simulink model "CanBusRagnar2020"  (R2021a)
settings: Solver=VariableStepAuto  StartTime=0.0  StopTime=10.0  RelTol=1e-3
model workspace (MAT data in the model file):
  A = [0  0  0  0  1  0  0  0; 0  0  0  0  0  1  0  0; 0  0  0  0  0  0  1  0; 0  0  0  0  0  0  0  1; 0  0  0  0  0  0  0  0; 0  0  0  0  0  0  0  0; 0  0  0  0  0  0  0  0; 0  0  0  0  0  0  0  0]
  Acl = [0  0  0  0  1  0  0  0  0  0  0  0  0  0  0  0; 0  0  0  0  0  1  0  0  0  0  0  0  0  0  0  0; 0  0  0  0  0  0  1  0  0  0  0  0  0  0  0  0; 0  0  0  0  0  0  0  1  0  0  0  0  0  0  0  0; 0  0  0  0  0  0  0  0  -1.14285714286  0  0  0  -2.14285714286  0  0  0; 0  0  0  0  0  0  0  0  0  -2.69387755102  0  0  0  -3.28571428571  0  0; 0  0  0  0  0  0  0  0  0  0  -2.38775510204  0  0  0  -3.14285714286  0; 0  0  0  0  0  0  0  0  0  0  0  -2.85714285714  0  0  0  -3.42857142857; 8.14285714286  0  0  0  0  0  0  0  -8.14285714286  0  0  0  1  0  0  0; 0  9.28571428571  0  0  0  0  0  0  0  -9.28571428571  0  0  0  1  0  0; 0  0  9.14285714286  0  0  0  0  0  0  0  -9.14285714286  0  0  0  1  0; 0  0  0  9.42857142857  0  0  0  0  0  0  0  -9.42857142857  0  0  0  1; 16.5714285714  0  0  0  0  0  0  0  -17.7142857143  0  0  0  -2.14285714286  0  0  0; 0  21.5510204082  0  0  0  0  0  0  0  -24.2448979592  0  0  0  -3.28571428571  0  0; 0  0  20.8163265306  0  0  0  0  0  0  0  -23.2040816327  0  0  0  -3.14285714286  0; 0  0  0  22.1428571429  0  0  0  0  0  0  0  -25  0  0  0  -3.42857142857]
  Ak_mimo = [-8.14285714286  0  0  0  1  0  0  0; 0  -9.28571428571  0  0  0  1  0  0; 0  0  -9.14285714286  0  0  0  1  0; 0  0  0  -9.42857142857  0  0  0  1; -17.7142857143  0  0  0  -2.14285714286  0  0  0; 0  -24.2448979592  0  0  0  -3.28571428571  0  0; 0  0  -23.2040816327  0  0  0  -3.14285714286  0; 0  0  0  -25  0  0  0  -3.42857142857]
  Ar = [0  0  0  0  1  0  0  0; 0  0  0  0  0  1  0  0; 0  0  0  0  0  0  1  0; 0  0  0  0  0  0  0  1; 0  0  0  0  0  0  0  0; 0  0  0  0  0  0  0  0; 0  0  0  0  0  0  0  0; 0  0  0  0  0  0  0  0]
  Aza = [-8.14285714286  0  0  0  1  0  0  0; 0  -9.28571428571  0  0  0  1  0  0; 0  0  -9.14285714286  0  0  0  1  0; 0  0  0  -9.42857142857  0  0  0  1; -17.7142857143  0  0  0  -2.14285714286  0  0  0; 0  -24.2448979592  0  0  0  -3.28571428571  0  0; 0  0  -23.2040816327  0  0  0  -3.14285714286  0; 0  0  0  -25  0  0  0  -3.42857142857]
  B = [0  0  0  0; 0  0  0  0; 0  0  0  0; 0  0  0  0; 0.78125  0  0  0; 0  0.78125  0  0; 0  0  0.78125  0; 0  0  0  2180]
  BScal = [0  0  0  0  0  0  0  0; 0  0  0  0  0  0  0  0; 0  0  0  0  0  0  0  0; 0  0  0  0  0  0  0  0; 0  0  0  0  0.78125  0  0  0; 0  0  0  0  0  0.78125  0  0; 0  0  0  0  0  0  0.78125  0; 0  0  0  0  0  0  0  2180]
  B_tilde_cl = [0  0  0  0; 0  0  0  0; 0  0  0  0; 0  0  0  0; 0.78125  0  0  0; 0  0.78125  0  0; 0  0  0.78125  0; 0  0  0  2180; 0.385570788906  0  0  0; 0  0.206011164513  0  0; 0  0  0.222133260428  0; 0  0  0  542.533936652; 2.03394557925  0  0  0; 0  1.56343339307  0  0; 0  0  1.60680460084  0; 0  0  0  4271.22171946]
  Bcl = [0  0  0  0; 0  0  0  0; 0  0  0  0; 0  0  0  0; 4.41904761905  0  0  0; 0  8.3179377014  0  0; 0  0  7.61096938775  0; 0  0  0  8.68347338936; 2.18093526616  0  0  0; 0  2.19339268123  0  0; 0  0  2.16403128975  0; 0  0  0  2.16104541364; 11.5047710326  0  0  0; 0  16.6458132017  0  0; 0  0  15.6535560053  0; 0  0  0  17.0133211656]
  Br = [0  0  0  0  0  0; 0  0  0  0  0  0; 0  0  0  0  0  0; 0  0  0  0  0  0; -1.78690965265  -1.76597744937  0.0707960973387  -0.101560505719  -0.0023778339261  -0.015199322583; -0.257428405219  0.0105056515104  0.812345370997  -0.775769674732  0.91789299065  1.98446037164; -1.43357477539  1.39250814302  0.227091277663  -0.200202188428  -0.464746757877  -1.31745089225; -116.29654411  106.543521913  161.685932847  -153.30180579  -42.3194853416  310.344292239]
  Br_test = [0  0  0  0  0  0; 0  0  0  0  0  0; 0  0  0  0  0  0; 0  0  0  0  0  0; -1.78690965265  -1.76597744937  0.0707960973387  -0.101560505719  -0.0023778339261  -0.015199322583; -0.257428405219  0.0105056515104  0.812345370997  -0.775769674732  0.91789299065  1.98446037164; -1.43357477539  1.39250814302  0.227091277663  -0.200202188428  -0.464746757877  -1.31745089225; -116.29654411  106.543521913  161.685932847  -153.30180579  -42.3194853416  310.344292239]
  C = [1  0  0  0  0  0  0  0; 0  1  0  0  0  0  0  0; 0  0  1  0  0  0  0  0; 0  0  0  1  0  0  0  0]
  CL_mimo = ss
  CL_mimo.IOSize_ = [4 4]
  CL_mimo.Data_ = ltipack.ssdata
  CL_mimo.Data_.a = [0  0  0  0  1  0  0  0  0  0  0  0  0  0  0  0; 0  0  0  0  0  1  0  0  0  0  0  0  0  0  0  0; 0  0  0  0  0  0  1  0  0  0  0  0  0  0  0  0; 0  0  0  0  0  0  0  1  0  0  0  0  0  0  0  0; 0  0  0  0  0  0  0  0  1.14285714286  0  0  0  2.14285714286  0  0  0; 0  0  0  0  0  0  0  0  0  2.69387755102  0  0  0  3.28571428571  0  0; 0  0  0  0  0  0  0  0  0  0  2.38775510204  0  0  0  3.14285714286  0; 0  0  0  0  0  0  0  0  0  0  0  2.85714285714  0  0  0  3.42857142857; -8.14285714286  0  0  0  0  0  0  0  -8.14285714286  0  0  0  1  0  0  0; 0  -9.28571428571  0  0  0  0  0  0  0  -9.28571428571  0  0  0  1  0  0; 0  0  -9.14285714286  0  0  0  0  0  0  0  -9.14285714286  0  0  0  1  0; 0  0  0  -9.42857142857  0  0  0  0  0  0  0  -9.42857142857  0  0  0  1; -16.5714285714  0  0  0  0  0  0  0  -17.7142857143  0  0  0  -2.14285714286  0  0  0; 0  -21.5510204082  0  0  0  0  0  0  0  -24.2448979592  0  0  0  -3.28571428571  0  0; 0  0  -20.8163265306  0  0  0  0  0  0  0  -23.2040816327  0  0  0  -3.14285714286  0; 0  0  0  -22.1428571429  0  0  0  0  0  0  0  -25  0  0  0  -3.42857142857]
  CL_mimo.Data_.b = [0  0  0  0; 0  0  0  0; 0  0  0  0; 0  0  0  0; 0.78125  0  0  0; 0  0.78125  0  0; 0  0  0.78125  0; 0  0  0  2180; 0  0  0  0; 0  0  0  0; 0  0  0  0; 0  0  0  0; 0  0  0  0; 0  0  0  0; 0  0  0  0; 0  0  0  0]
  CL_mimo.Data_.c = [1  0  0  0  0  0  0  0  0  0  0  0  0  0  0  0; 0  1  0  0  0  0  0  0  0  0  0  0  0  0  0  0; 0  0  1  0  0  0  0  0  0  0  0  0  0  0  0  0; 0  0  0  1  0  0  0  0  0  0  0  0  0  0  0  0]
  CL_mimo.Data_.d = [0  0  0  0; 0  0  0  0; 0  0  0  0; 0  0  0  0]
  CL_mimo.Data_.Delay.Input = [0; 0; 0; 0]
  CL_mimo.Data_.Delay.Output = [0; 0; 0; 0]
  CL_mimo.Data_.Delay.Internal = []
  CL_mimo.Data_.Ts = 0
  CLpoles_Mimo = [-1; -1.14285714286; -4; -4.14285714286; -5; -4.85714285714; -4.71428571429; -4.57142857143; -4.28571428571; -4.42857142857; -1.28571428571; -2; -1.85714285714; -1.71428571429; -1.42857142857; -1.57142857143]
  Ccl = [1  0  0  0  0  0  0  0  0  0  0  0  0  0  0  0; 0  1  0  0  0  0  0  0  0  0  0  0  0  0  0  0; 0  0  1  0  0  0  0  0  0  0  0  0  0  0  0  0; 0  0  0  1  0  0  0  0  0  0  0  0  0  0  0  0]
  Cr = [-0.206927442386  -0.0944061499718  -0.216271921634  -0.0415455690518  0  0  0  0; -0.232824651508  0.102097811543  0.225597256187  0.111631735372  0  0  0  0; -0.00180373943386  0.0780892312781  0.0597928263858  0.966089378788  0  0  0  0; -0.00272377706545  -0.0720989537283  -0.0538834160618  -0.939605746145  0  0  0  0; -0.0466166768285  0.780547176224  0.236218176976  -11.3071111582  0  0  0  0; -0.00437482668944  -0.0402889466393  -0.184050607434  4.46123014123  0  0  0  0]
  Cza = [1.46285714286  0  0  0  2.74285714286  0  0  0; 0  3.44816326531  0  0  0  4.20571428571  0  0; 0  0  3.05632653061  0  0  0  4.02285714286  0; 0  0  0  0.00131061598952  0  0  0  0.00157273918742]
  D = [0  0  0  0  0  0; 0  0  0  0  0  0; 0  0  0  0  0  0; 0  0  0  0  0  0]
  Desired_poles = [-2 -1.85714285714 -1.71428571429 -1.57142857143 -1.42857142857 -1.28571428571 -1.14285714286 -1]
  Desired_poles_obs = [-5 -4.85714285714 -4.71428571429 -4.57142857143 -4.42857142857 -4.28571428571 -4.14285714286 -4]
  Desired_zeroes = [-3 -2.85714285714 -2.71428571429 -2.57142857143 -2.42857142857 -2.28571428571 -2.14285714286 -2]
  Dr = [0  0  0  0  0  0; 0  0  0  0  0  0; 0  0  0  0  0  0; 0  0  0  0  0  0]
  F = [-1.46285714286  0  0  0  -2.74285714286  0  0  0; 0  -3.44816326531  0  0  0  -4.20571428571  0  0; 0  0  -3.05632653061  0  0  0  -4.02285714286  0; 0  0  0  -0.00131061598952  0  0  0  -0.00157273918742]
  F_mimo = [-1.46285714286  0  0  0  -2.74285714286  0  0  0; 0  -3.44816326531  0  0  0  -4.20571428571  0  0; 0  0  -3.05632653061  0  0  0  -4.02285714286  0; 0  0  0  -0.00131061598952  0  0  0  -0.00157273918742]
  J = [-0.206927442386  -0.232824651508  -0.00180373943386  -0.00272377706545  -0.0466166768285  -0.00437482668944; -0.0944061499718  0.102097811543  0.0780892312781  -0.0720989537283  0.780547176224  -0.0402889466393; -0.216271921634  0.225597256187  0.0597928263858  -0.0538834160618  0.236218176976  -0.184050607434; -0.0415455690518  0.111631735372  0.966089378788  -0.939605746145  -11.3071111582  4.46123014123]
  Joint_op = [1.0187; 2.0405; 0.0915; 2.9254; 0.58469; 0.62011]
  L = [-8.14285714286  0  0  0; 0  -9.28571428571  0  0; 0  0  -9.14285714286  0; 0  0  0  -9.42857142857; -16.5714285714  0  0  0; 0  -21.5510204082  0  0; 0  0  -20.8163265306  0; 0  0  0  -22.1428571429]
  L_mimo = [-8.14285714286  0  0  0; 0  -9.28571428571  0  0; 0  0  -9.14285714286  0; 0  0  0  -9.42857142857; -16.5714285714  0  0  0; 0  -21.5510204082  0  0; 0  0  -20.8163265306  0; 0  0  0  -22.1428571429]
  M = [2.18093526616  0  0  0; 0  2.19339268123  0  0; 0  0  2.16403128975  0; 0  0  0  2.16104541364; 11.5047710326  0  0  0; 0  16.6458132017  0  0; 0  0  15.6535560053  0; 0  0  0  17.0133211656]
  M_tilde = [0.385570788906  0  0  0; 0  0.206011164513  0  0; 0  0  0.222133260428  0; 0  0  0  542.533936652; 2.03394557925  0  0  0; 0  1.56343339307  0  0; 0  0  1.60680460084  0; 0  0  0  4271.22171946]
  MassM = [0.78125  0  0  0; 0  0.78125  0  0; 0  0  0.78125  0; 0  0  0  2180]
  N = [5.65638095238  0  0  0; 0  10.6469602578  0  0; 0  0  9.74204081633  0; 0  0  0  0.00398324467402]
  Q = [-0.161662064364  -0.0737548046654  -0.168962438777  -90.569340533; -0.181894258991  0.0797639152681  0.176247856396  243.357183112; -0.00140917143271  0.061007211936  0.0467131456139  2106.07484576; -0.00212795083238  -0.0563273076002  -0.0420964187983  -2048.3405266; -0.0364192787723  0.609802481425  0.184545450762  -24649.502325; -0.00341783335112  -0.031475739562  -0.143789537058  9725.48170789]
  Ragnar_JS = ss
  Ragnar_JS.IOSize_ = [6 6]
  Ragnar_JS.Data_ = ltipack.ssdata
  Ragnar_JS.Data_.a = [0  0  0  0  1  0  0  0; 0  0  0  0  0  1  0  0; 0  0  0  0  0  0  1  0; 0  0  0  0  0  0  0  1; 0  0  0  0  0  0  0  0; 0  0  0  0  0  0  0  0; 0  0  0  0  0  0  0  0; 0  0  0  0  0  0  0  0]
  Ragnar_JS.Data_.b = [0  0  0  0  0  0; 0  0  0  0  0  0; 0  0  0  0  0  0; 0  0  0  0  0  0; -1.78690965265  -1.76597744937  0.0707960973387  -0.101560505719  -0.0023778339261  -0.015199322583; -0.257428405219  0.0105056515104  0.812345370997  -0.775769674732  0.91789299065  1.98446037164; -1.43357477539  1.39250814302  0.227091277663  -0.200202188428  -0.464746757877  -1.31745089225; -116.29654411  106.543521913  161.685932847  -153.30180579  -42.3194853416  310.344292239]
  Ragnar_JS.Data_.c = [-0.206927442386  -0.0944061499718  -0.216271921634  -0.0415455690518  0  0  0  0; -0.232824651508  0.102097811543  0.225597256187  0.111631735372  0  0  0  0; -0.00180373943386  0.0780892312781  0.0597928263858  0.966089378788  0  0  0  0; -0.00272377706545  -0.0720989537283  -0.0538834160618  -0.939605746145  0  0  0  0; -0.0466166768285  0.780547176224  0.236218176976  -11.3071111582  0  0  0  0; -0.00437482668944  -0.0402889466393  -0.184050607434  4.46123014123  0  0  0  0]
  Ragnar_JS.Data_.d = [0  0  0  0  0  0; 0  0  0  0  0  0; 0  0  0  0  0  0; 0  0  0  0  0  0; 0  0  0  0  0  0; 0  0  0  0  0  0]
  Ragnar_JS.Data_.Delay.Input = [0; 0; 0; 0; 0; 0]
  Ragnar_JS.Data_.Delay.Output = [0; 0; 0; 0; 0; 0]
  Ragnar_JS.Data_.Delay.Internal = []
  Ragnar_JS.Data_.Ts = 0
  Sig = Simulink.Signal
  Sig.DataType = 'auto'
  Sig.Dimensions = -1
  Sig.DimensionsMode = 'auto'
  Sig.Complexity = 'auto'
  Sig.SampleTime = -1
  Sig.SamplingMode = 'auto'
  Task_op = [0; 0.5; -0.4; 1.57079632679]
  final_sys = ss
  final_sys.IOSize_ = [4 4]
  final_sys.Data_ = ltipack.ssdata
  final_sys.Data_.a = [0  0  0  0  1  0  0  0  0  0  0  0  0  0  0  0; 0  0  0  0  0  1  0  0  0  0  0  0  0  0  0  0; 0  0  0  0  0  0  1  0  0  0  0  0  0  0  0  0; 0  0  0  0  0  0  0  1  0  0  0  0  0  0  0  0; 0  0  0  0  0  0  0  0  -1.14285714286  0  0  0  -2.14285714286  0  0  0; 0  0  0  0  0  0  0  0  0  -2.69387755102  0  0  0  -3.28571428571  0  0; 0  0  0  0  0  0  0  0  0  0  -2.38775510204  0  0  0  -3.14285714286  0; 0  0  0  0  0  0  0  0  0  0  0  -2.85714285714  0  0  0  -3.42857142857; 8.14285714286  0  0  0  0  0  0  0  -8.14285714286  0  0  0  1  0  0  0; 0  9.28571428571  0  0  0  0  0  0  0  -9.28571428571  0  0  0  1  0  0; 0  0  9.14285714286  0  0  0  0  0  0  0  -9.14285714286  0  0  0  1  0; 0  0  0  9.42857142857  0  0  0  0  0  0  0  -9.42857142857  0  0  0  1; 16.5714285714  0  0  0  0  0  0  0  -17.7142857143  0  0  0  -2.14285714286  0  0  0; 0  21.5510204082  0  0  0  0  0  0  0  -24.2448979592  0  0  0  -3.28571428571  0  0; 0  0  20.8163265306  0  0  0  0  0  0  0  -23.2040816327  0  0  0  -3.14285714286  0; 0  0  0  22.1428571429  0  0  0  0  0  0  0  -25  0  0  0  -3.42857142857]
  final_sys.Data_.b = [0  0  0  0; 0  0  0  0; 0  0  0  0; 0  0  0  0; 4.41904761905  0  0  0; 0  8.3179377014  0  0; 0  0  7.61096938775  0; 0  0  0  8.68347338936; 2.18093526616  0  0  0; 0  2.19339268123  0  0; 0  0  2.16403128975  0; 0  0  0  2.16104541364; 11.5047710326  0  0  0; 0  16.6458132017  0  0; 0  0  15.6535560053  0; 0  0  0  17.0133211656]
  final_sys.Data_.c = [1  0  0  0  0  0  0  0  0  0  0  0  0  0  0  0; 0  1  0  0  0  0  0  0  0  0  0  0  0  0  0  0; 0  0  1  0  0  0  0  0  0  0  0  0  0  0  0  0; 0  0  0  1  0  0  0  0  0  0  0  0  0  0  0  0]
  final_sys.Data_.d = [0  0  0  0; 0  0  0  0; 0  0  0  0; 0  0  0  0]
  final_sys.Data_.Delay.Input = [0; 0; 0; 0]
  final_sys.Data_.Delay.Output = [0; 0; 0; 0]
  final_sys.Data_.Delay.Internal = []
  final_sys.Data_.Ts = 0
  out = Simulink.SimulationOutput
  out.Data.tout = [0; 3.15544362088e-30; 0.005; 0.005; 0.005; 0.0050512; 0.0050512; 0.0050512; 0.0050512; 0.0051024; 0.0051024; 0.0051024; 0.0051536; 0.0051536; 0.0052048; 0.0052048; 0.005256; 0.005256; 0.005256; 0.0053072; 0.0053072; 0.0053584; 0.0053584; 0.0053584; 0.0054096; 0.0054608; 0.0055632; 0.005768; 0.0061776; 0.0069968; 0.00863519999999; 0.0100512; 0.0100512; 0.0101024]
  out.Metadata = Simulink.SimulationMetadata
  out.Metadata.ModelInfo.ModelName = 'CanBusRagnar2020'
  out.Metadata.ModelInfo.ModelVersion = '2.3'
  out.Metadata.ModelInfo.ModelFilePath = 'C:\Users\mozzr\Documents\control-courses\CanBusRagnar\CanBusRagnar2020.slx'
  out.Metadata.ModelInfo.UserID = 'mozzr'
  out.Metadata.ModelInfo.MachineName = 'DESKTOP-FJO0ONK'
  out.Metadata.ModelInfo.Platform = 'PCWIN64'
  out.Metadata.ModelInfo.ModelStructuralChecksum = [687622235; 3512854413; 2358566999; 3204458558]
  out.Metadata.ModelInfo.SimulationMode = 'normal'
  out.Metadata.ModelInfo.StartTime = 0
  out.Metadata.ModelInfo.StopTime = 0.0101024
  out.Metadata.ModelInfo.SolverInfo.Type = 'Variable-Step'
  out.Metadata.ModelInfo.SolverInfo.Solver = 'ode45'
  out.Metadata.ModelInfo.SolverInfo.MaxStepSize = 0.2
  out.Metadata.ModelInfo.SimulinkVersion.Name = 'Simulink'
  out.Metadata.ModelInfo.SimulinkVersion.Version = '10.3'
  out.Metadata.ModelInfo.SimulinkVersion.Release = '(R2021a)'
  out.Metadata.ModelInfo.SimulinkVersion.Date = '14-Nov-2020'
  out.Metadata.ModelInfo.LoggingInfo.LoggingToFile = 'off'
  out.Metadata.TimingInfo.WallClockTimestampStart = '2021-11-10 14:43:59'
  out.Metadata.TimingInfo.WallClockTimestampStop = '2021-11-10 14:44:00'
  out.Metadata.TimingInfo.InitializationElapsedWallTime = 0.4461101
  out.Metadata.TimingInfo.ExecutionElapsedWallTime = 0.1552773
  out.Metadata.TimingInfo.TerminationElapsedWallTime = 0.056487
  out.Metadata.TimingInfo.TotalElapsedWallTime = 0.6578744
  out.Metadata.TimingInfo.ProfilerData = 'Profiler is not enabled'
  out.Metadata.ExecutionInfo.StopEvent = 'DiagnosticError'
  out.Metadata.ExecutionInfo.StopEventSource = []
  out.Metadata.ExecutionInfo.StopEventDescription = 'Error occurred in ''<a href="matlab:open_and_hilite_hyperlink (''CanBusRagnar2020/TrueTime Kernel (Teensy)'',''error'')">CanBusRagnar2020/TrueTime Kernel (Teensy)</a>''. Unrecognized function or variable ''Task_op''.'
  out.Metadata.ExecutionInfo.ErrorDiagnostic.Diagnostic = MSLDiagnostic
  out.Metadata.ExecutionInfo.ErrorDiagnostic.Diagnostic.identifier = 'Simulink:blocks:SubsysErrFcnMsg'
  out.Metadata.ExecutionInfo.ErrorDiagnostic.Diagnostic.message = 'Error occurred in ''<a href="matlab:open_and_hilite_hyperlink (''CanBusRagnar2020/TrueTime Kernel (Teensy)'',''error'')">CanBusRagnar2020/TrueTime Kernel (Teensy)</a>''. Unrecognized function or variable ''Task_op''.'
  out.Metadata.ExecutionInfo.ErrorDiagnostic.Diagnostic.paths = {'CanBusRagnar2020/TrueTime Kernel (Teensy)'}
  out.Metadata.ExecutionInfo.ErrorDiagnostic.Diagnostic.cause{1} = MSLDiagnostic
  out.Metadata.ExecutionInfo.ErrorDiagnostic.Diagnostic.cause{1}.identifier = 'Simulink:blocks:SubsysErrFcnMsg'
  out.Metadata.ExecutionInfo.ErrorDiagnostic.Diagnostic.cause{1}.message = 'Error occurred in ''CanBusRagnar2020/TrueTime Kernel (Teensy)''. Unrecognized function or variable ''Task_op''.'
  out.Metadata.ExecutionInfo.ErrorDiagnostic.Diagnostic.cause{1}.paths = {'CanBusRagnar2020/TrueTime Kernel (Teensy)'}
  out.Metadata.ExecutionInfo.ErrorDiagnostic.Diagnostic.cause{1}.arguments = {'CanBusRagnar2020/TrueTime Kernel (Teensy)', 'Unrecognized function or variable ''Task_op''.'}
  out.Metadata.ExecutionInfo.ErrorDiagnostic.Diagnostic.cause{1}.stack = struct([])
  out.Metadata.ExecutionInfo.ErrorDiagnostic.Diagnostic.cause{1}.metaDataProp.UI = []
  out.Metadata.ExecutionInfo.ErrorDiagnostic.Diagnostic.cause{1}.metaDataProp.STAGE = []
  out.Metadata.ExecutionInfo.ErrorDiagnostic.Diagnostic.cause{1}.metaDataProp.CATEGORY = []
  out.Metadata.ExecutionInfo.ErrorDiagnostic.Diagnostic.cause{1}.metaDataProp.COMPONENT = []
  out.Metadata.ExecutionInfo.ErrorDiagnostic.Diagnostic.cause{1}.metaDataProp.MDL_NAME = []
  out.Metadata.ExecutionInfo.ErrorDiagnostic.Diagnostic.cause{1}.metaDataProp.ACTION = ''
  out.Metadata.ExecutionInfo.ErrorDiagnostic.Diagnostic.cause{1}.metaDataProp.DOC = []
  out.Metadata.ExecutionInfo.ErrorDiagnostic.Diagnostic.cause{1}.metaDataProp.SUB_CATEGORY = []
  out.Metadata.ExecutionInfo.ErrorDiagnostic.Diagnostic.cause{1}.metaDataProp.MSTACK_PRESERVE = []
  out.Metadata.ExecutionInfo.ErrorDiagnostic.Diagnostic.cause{1}.metaDataProp.DOUBLE_ARGS = []
  out.Metadata.ExecutionInfo.ErrorDiagnostic.Diagnostic.arguments = {'CanBusRagnar2020/TrueTime Kernel (Teensy)', 'Unrecognized function or variable ''Task_op''.'}
  out.Metadata.ExecutionInfo.ErrorDiagnostic.Diagnostic.stack = struct([])
  out.Metadata.ExecutionInfo.ErrorDiagnostic.Diagnostic.metaDataProp.UI = []
  out.Metadata.ExecutionInfo.ErrorDiagnostic.Diagnostic.metaDataProp.STAGE = []
  out.Metadata.ExecutionInfo.ErrorDiagnostic.Diagnostic.metaDataProp.CATEGORY = []
  out.Metadata.ExecutionInfo.ErrorDiagnostic.Diagnostic.metaDataProp.COMPONENT = []
  out.Metadata.ExecutionInfo.ErrorDiagnostic.Diagnostic.metaDataProp.MDL_NAME = []
  out.Metadata.ExecutionInfo.ErrorDiagnostic.Diagnostic.metaDataProp.ACTION = ''
  out.Metadata.ExecutionInfo.ErrorDiagnostic.Diagnostic.metaDataProp.DOC = []
  out.Metadata.ExecutionInfo.ErrorDiagnostic.Diagnostic.metaDataProp.SUB_CATEGORY = []
  out.Metadata.ExecutionInfo.ErrorDiagnostic.Diagnostic.metaDataProp.MSTACK_PRESERVE = []
  out.Metadata.ExecutionInfo.ErrorDiagnostic.Diagnostic.metaDataProp.DOUBLE_ARGS = []
  out.Metadata.ExecutionInfo.ErrorDiagnostic.SimulationPhase = 'Execution'
  out.Metadata.ExecutionInfo.ErrorDiagnostic.SimulationTime = 0.0101024
  out.Metadata.ExecutionInfo.WarningDiagnostics = struct([])
  out.Metadata.AppInfo = struct()
  out.ErrorMessage = 'Error occurred in ''<a href="matlab:open_and_hilite_hyperlink (''CanBusRagnar2020/TrueTime Kernel (Teensy)'',''error'')">CanBusRagnar2020/TrueTime Kernel (Teensy)</a>''. Unrecognized function or variable ''Task_op''.
    | Caused by:
    |     Error occurred in ''CanBusRagnar2020/TrueTime Kernel (Teensy)''. Unrecognized function or variable ''Task_op''.'
  sys_k_mimo = ss
  sys_k_mimo.IOSize_ = [4 4]
  sys_k_mimo.Data_ = ltipack.ssdata
  sys_k_mimo.Data_.a = [-8.14285714286  0  0  0  1  0  0  0; 0  -9.28571428571  0  0  0  1  0  0; 0  0  -9.14285714286  0  0  0  1  0; 0  0  0  -9.42857142857  0  0  0  1; -17.7142857143  0  0  0  -2.14285714286  0  0  0; 0  -24.2448979592  0  0  0  -3.28571428571  0  0; 0  0  -23.2040816327  0  0  0  -3.14285714286  0; 0  0  0  -25  0  0  0  -3.42857142857]
  sys_k_mimo.Data_.b = [-8.14285714286  0  0  0; 0  -9.28571428571  0  0; 0  0  -9.14285714286  0; 0  0  0  -9.42857142857; -16.5714285714  0  0  0; 0  -21.5510204082  0  0; 0  0  -20.8163265306  0; 0  0  0  -22.1428571429]
  sys_k_mimo.Data_.c = [1.46285714286  0  0  0  2.74285714286  0  0  0; 0  3.44816326531  0  0  0  4.20571428571  0  0; 0  0  3.05632653061  0  0  0  4.02285714286  0; 0  0  0  0.00131061598952  0  0  0  0.00157273918742]
  sys_k_mimo.Data_.d = [0  0  0  0; 0  0  0  0; 0  0  0  0; 0  0  0  0]
  sys_k_mimo.Data_.Delay.Input = [0; 0; 0; 0]
  sys_k_mimo.Data_.Delay.Output = [0; 0; 0; 0]
  sys_k_mimo.Data_.Delay.Internal = []
  sys_k_mimo.Data_.Ts = 0
  sys_mimo = ss
  sys_mimo.IOSize_ = [4 4]
  sys_mimo.Data_ = ltipack.ssdata
  sys_mimo.Data_.a = [0  0  0  0  1  0  0  0; 0  0  0  0  0  1  0  0; 0  0  0  0  0  0  1  0; 0  0  0  0  0  0  0  1; 0  0  0  0  0  0  0  0; 0  0  0  0  0  0  0  0; 0  0  0  0  0  0  0  0; 0  0  0  0  0  0  0  0]
  sys_mimo.Data_.b = [0  0  0  0; 0  0  0  0; 0  0  0  0; 0  0  0  0; 0.78125  0  0  0; 0  0.78125  0  0; 0  0  0.78125  0; 0  0  0  2180]
  sys_mimo.Data_.c = [1  0  0  0  0  0  0  0; 0  1  0  0  0  0  0  0; 0  0  1  0  0  0  0  0; 0  0  0  1  0  0  0  0]
  sys_mimo.Data_.d = [0  0  0  0; 0  0  0  0; 0  0  0  0; 0  0  0  0]
  sys_mimo.Data_.Delay.Input = [0; 0; 0; 0]
  sys_mimo.Data_.Delay.Output = [0; 0; 0; 0]
  sys_mimo.Data_.Delay.Internal = []
  sys_mimo.Data_.Ts = 0
libraries: truetime x8
settings Model: Creator=mozzr  LastModifiedBy=mozzr
settings SolverCC: AlgebraicLoopSolver=TrustRegion

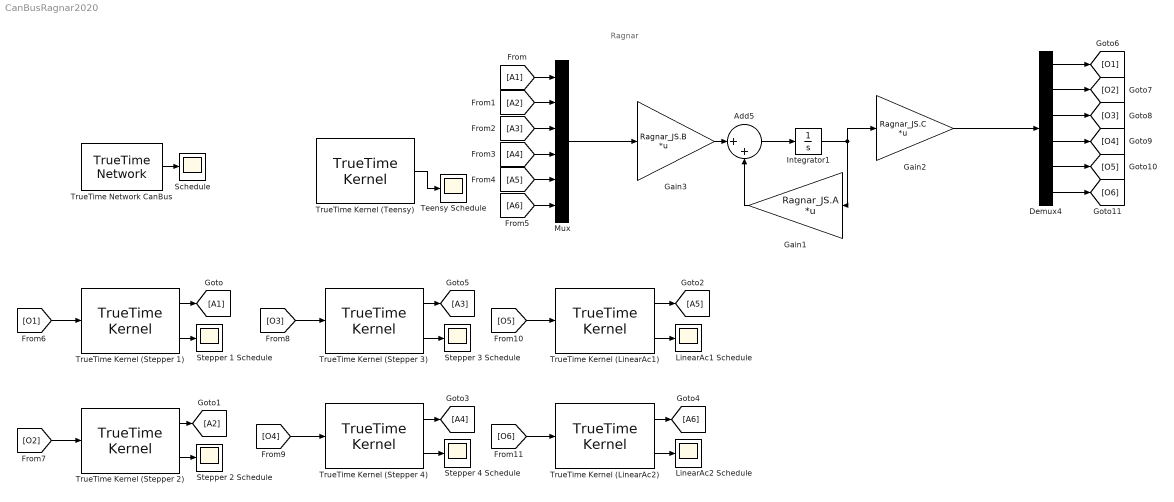
== system CanBusRagnar2020 ==
  note: Ragnar
  Add5 : Sum  Inputs=|++
  Demux4 : Demux  Outputs=6
  Gain1 : Gain  Gain=Ragnar_JS.A  Multiplication=Matrix(K*u)
  Gain2 : Gain  Gain=Ragnar_JS.C  Multiplication=Matrix(K*u)
  Gain3 : Gain  Gain=Ragnar_JS.B  Multiplication=Matrix(K*u)
  Integrator1 : Integrator
  LinearAc1 Schedule : Scope
  LinearAc2 Schedule : Scope
  Mux : Mux  Inputs=6
  Schedule : Scope
  Stepper 1 Schedule : Scope
  Stepper 2 Schedule : Scope
  Stepper 3 Schedule : Scope
  Stepper 4 Schedule : Scope
  Teensy Schedule : Scope
  TrueTime Kernel (LinearAc1) : truetime/TrueTime Kernel  sfun=LinearAc1_init  args=[]  ninputsoutputs=[1 1]  ntriggers=0  trigtype=falling  nwnodenbr=[1 6]  clockoffsetdrift=[0 0]  schedoutput=on  battery=off  poweroutput=off  label=1: 6
  TrueTime Kernel (LinearAc2) : truetime/TrueTime Kernel  sfun=LinearAc2_init  args=[]  ninputsoutputs=[1 1]  ntriggers=0  trigtype=falling  nwnodenbr=[1 7]  clockoffsetdrift=[0 0]  schedoutput=on  battery=off  poweroutput=off  label=1: 7
  TrueTime Kernel (Stepper 1) : truetime/TrueTime Kernel  sfun=Stepper1_init  args=[]  ninputsoutputs=[1 1]  ntriggers=0  trigtype=falling  nwnodenbr=[1 2]  clockoffsetdrift=[0 0]  schedoutput=on  battery=off  poweroutput=off  label=1: 2
  TrueTime Kernel (Stepper 2) : truetime/TrueTime Kernel  sfun=Stepper2_init  args=[]  ninputsoutputs=[1 1]  ntriggers=0  trigtype=falling  nwnodenbr=[1 3]  clockoffsetdrift=[0 0]  schedoutput=on  battery=off  poweroutput=off  label=1: 3
  TrueTime Kernel (Stepper 3) : truetime/TrueTime Kernel  sfun=Stepper3_init  args=[]  ninputsoutputs=[1 1]  ntriggers=0  trigtype=falling  nwnodenbr=[1 4]  clockoffsetdrift=[0 0]  schedoutput=on  battery=off  poweroutput=off  label=1: 4
  TrueTime Kernel (Stepper 4) : truetime/TrueTime Kernel  sfun=Stepper4_init  args=[]  ninputsoutputs=[1 1]  ntriggers=0  trigtype=falling  nwnodenbr=[1 5]  clockoffsetdrift=[0 0]  schedoutput=on  battery=off  poweroutput=off  label=1: 5
  TrueTime Kernel (Teensy) : truetime/TrueTime Kernel  sfun=Teensy_init  args=[]  ninputsoutputs=[0 0]  ntriggers=0  trigtype=falling  nwnodenbr=[1 1]  clockoffsetdrift=[0 0]  schedoutput=on  battery=off  poweroutput=off  label=1: 1
  TrueTime Network CanBus : truetime/TrueTime Network  nwtype=CSMA/AMP (CAN)  nwnbr=1  nnodes=7  rate=10000000  minsize=512  lossprob=0  seed=0  bandwidths=[0.5 0.5]  slotsize=512  schedule=[1 1 2]  memsize=80000  buftype=Common buffer  overflow=Retransmit  dynSchedule=0  miniSlotSize=0  NIT=0  QSortMode=FIFO  sync=0  irtSchedule=0  nrtLength=0  nodeGraph=0  scheduleoutput=on
  wires:
  TrueTime Kernel (Stepper 2)/2 -> Stepper 2 Schedule/1
  TrueTime Kernel (Stepper 1)/2 -> Stepper 1 Schedule/1
  TrueTime Kernel (Stepper 4)/2 -> Stepper 4 Schedule/1
  TrueTime Kernel (Stepper 3)/2 -> Stepper 3 Schedule/1
  TrueTime Kernel (LinearAc1)/2 -> LinearAc1 Schedule/1
  TrueTime Kernel (LinearAc2)/2 -> LinearAc2 Schedule/1
  TrueTime Kernel (Teensy)/1 -> Teensy Schedule/1
  TrueTime Network CanBus/1 -> Schedule/1
  Gain2/1 -> Demux4/1
  Gain1/1 -> Add5/2
  Integrator1/1 -> Gain1/1, Gain2/1
  Add5/1 -> Integrator1/1
  Gain3/1 -> Add5/1
  TrueTime Kernel (Stepper 1)/1 -> [A1]
  [A1] -> Mux/1
  TrueTime Kernel (Stepper 2)/1 -> [A2]
  TrueTime Kernel (LinearAc1)/1 -> [A5]
  TrueTime Kernel (Stepper 4)/1 -> [A4]
  TrueTime Kernel (LinearAc2)/1 -> [A6]
  TrueTime Kernel (Stepper 3)/1 -> [A3]
  [A2] -> Mux/2
  [A3] -> Mux/3
  [A4] -> Mux/4
  [A5] -> Mux/5
  [A6] -> Mux/6
  Mux/1 -> Gain3/1
  Demux4/1 -> [O1]
  Demux4/2 -> [O2]
  Demux4/3 -> [O3]
  Demux4/4 -> [O4]
  Demux4/5 -> [O5]
  Demux4/6 -> [O6]
  [O1] -> TrueTime Kernel (Stepper 1)/1
  [O2] -> TrueTime Kernel (Stepper 2)/1
  [O3] -> TrueTime Kernel (Stepper 3)/1
  [O4] -> TrueTime Kernel (Stepper 4)/1
  [O5] -> TrueTime Kernel (LinearAc1)/1
  [O6] -> TrueTime Kernel (LinearAc2)/1
